simulink model "force_control_teaching_harness"  (R2016b)
settings: Solver=ode45  StartTime=0.0  StopTime=1  RelTol=1e-3  EnableMultiTasking=on
undefined symbols (not defined in the file): sigbuilder_block
settings Model: ModifiedByFormat=The MathWorks Inc.  Creator=The MathWorks, Inc.  LastModifiedBy=The MathWorks Inc.
settings DataIOCC: LimitDataPoints=on  SaveFormat=Array  SaveOutput=off  SaveTime=off
settings OptimizationCC: ExpressionDepthLimit=2147483647  LifeSpan=1
settings DebuggingCC: UnderspecifiedInitializationDetection=Classic  MergeDetectMultiDrivingBlocksExec=none  SolverPrmCheckMsg=warning  FcnCallInpInsideContextMsg=warning  StateNameClashWarn=warning  SFUnexpectedBacktrackingDiag=warning  SFNoUnconditionalDefaultTransitionDiag=warning  SFExecutionAtInitializationDiag=none
settings HardwareCC: ProdBitPerPointer=32  ProdBitPerSizeT=32  ProdBitPerPtrDiffT=32  ProdLargestAtomicFloat=None  ProdIntDivRoundTo=Undefined  ProdEndianess=Unspecified  ProdWordSize=32  ProdHWDeviceType=32-bit Generic
settings ModelReferenceCC: PropagateSignalLabelsOutOfModel=off
settings GRTTargetCC: TargetLangStandard=C89/C90 (ANSI)  GeneratePreprocessorConditionals=Disable all  CombineOutputUpdateFcns=off  GRTInterface=on
settings ConfigComp: CovMetricSettings=dw  CovHtmlReporting=on  CovSaveCumulativeToWorkspaceVar=on  CovSaveSingleToWorkspaceVar=on  CovExternalEMLEnable=off  CovSFcnEnable=off

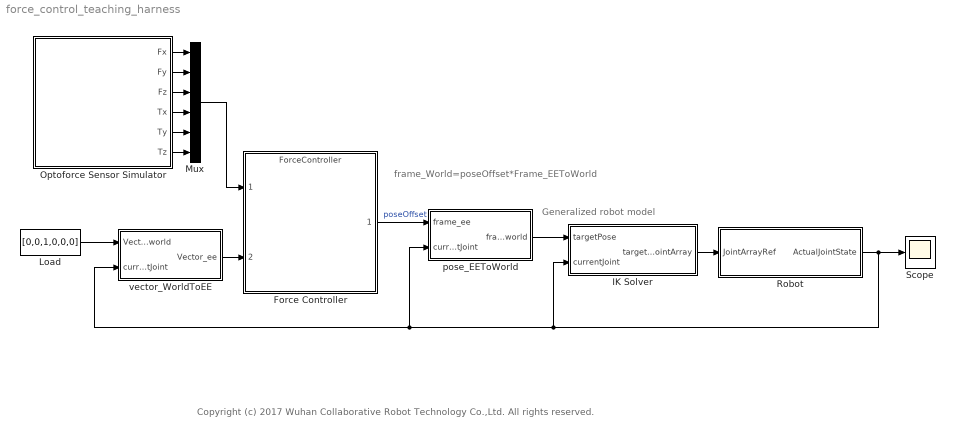
== system force_control_teaching_harness ==
  note: frame_World=poseOffset*Frame_EEToWorld
  note: Generalized robot model
  note: Copyright (c) 2017 Wuhan Collaborative Robot Technology Co.,Ltd. All rights reserved.
  Force Controller : ModelReference  ModelNameDialog=ForceController.slx  SimulationMode=Normal  ModelReferenceVersion=1.135
  IK Solver : Subsystem
  Load : Constant  Value=[0,0,1,0,0,0]
  Mux : Mux  Inputs=6
  Optoforce Sensor Simulator : Subsystem  Tag=STV Subsys  LoadFcn=sigbuilder_block('load');  StartFcn=sigbuilder_block('start');  StopFcn=sigbuilder_block('stop');  ClipboardFcn=sigbuilder_block('clipboard');  mask(Sigbuilder block){tuvar=[0:10]}
      mask help: Simulink:masks:SigbuilderBlock_MD
      mask init:
      | if ~strcmp(get_param(bdroot(gcbh),'SimulationStatus'),'stopped') tuvar = sigbuilder_block('maskInit'); end
      settings: CopyFcn=sigbuilder_block('copy');  DeleteFcn=sigbuilder_block('delete');  ModelCloseFcn=sigbuilder_block('modelClose');  PreSaveFcn=sigbuilder_block('preSave');  PauseFcn=sigbuilder_block('pause');  ContinueFcn=sigbuilder_block('continue');  NameChangeFcn=sigbuilder_block('namechange');  OpenFcn=sigbuilder_block('open',[6 30 1428 681 ]);  CloseFcn=sigbuilder_block('close');
      mask Display: plot(0, 0, 100, 100,[2, 2, 32, 32, 2], [68, 8, 8, 68, 68],[32, 2], [38, 38], [32, 19, 2],[53, 60, 44], [32, 17, 17, 2],[16, 16, 31, 31]);txt = getActiveGroup(gcbh);text(2, 100, txt,'verticalAlignment', 'top');
  Robot : Subsystem
  Scope : Scope
  pose_EEToWorld : Subsystem
  vector_WorldToEE : Subsystem
  wires:
  Optoforce Sensor Simulator/1(Fx) -> Mux/1
  Force Controller/1 -> pose_EEToWorld/1(frame_ee)  "poseOffset"
  Robot/1(ActualJointState) -> Scope/1, pose_EEToWorld/2(currentJoint), vector_WorldToEE/2(currentJoint), IK Solver/2(currentJoint)
  IK Solver/1(targetJointArray) -> Robot/1(JointArrayRef)
  Optoforce Sensor Simulator/2(Fy) -> Mux/2
  Optoforce Sensor Simulator/3(Fz) -> Mux/3
  Optoforce Sensor Simulator/4(Tx) -> Mux/4
  Optoforce Sensor Simulator/5(Ty) -> Mux/5
  Optoforce Sensor Simulator/6(Tz) -> Mux/6
  Mux/1 -> Force Controller/1
  Load/1 -> vector_WorldToEE/1(Vector_world)
  vector_WorldToEE/1(Vector_ee) -> Force Controller/2
  pose_EEToWorld/1(frame_world) -> IK Solver/1(targetPose)

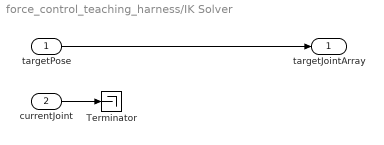
== system force_control_teaching_harness/IK Solver ==
  targetPose : Inport  PortDimensions=6
  currentJoint : Inport  Port=2  PortDimensions=6
  Terminator : Terminator
  targetJointArray : Outport
  wires:
  targetPose/1 -> targetJointArray/1
  currentJoint/1 -> Terminator/1

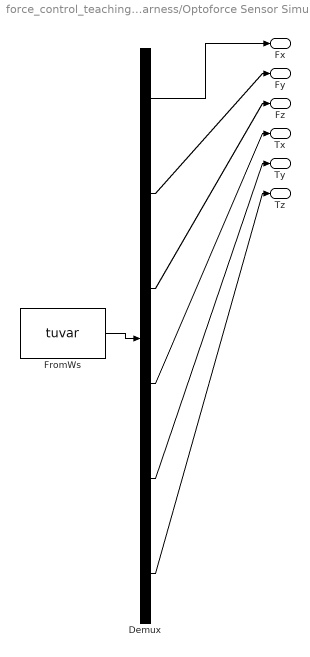
== system force_control_teaching_harness/Optoforce Sensor Simulator ==
  Demux : Demux  Tag=STV Demux  Outputs=6
  FromWs : FromWorkspace  Tag=STV FromWs  VariableName=tuvar  SampleTime=0
      SigBuilderData=|
      | common.afterFinalStr = 'Extrapolate'
      | common.sampleTime = 0
      | dataSet.timeRange = [0 10]
      | dataSet.name = 'Group 1'
      | sbobj.Groups.Name = 'Group 1'
      | sbobj.Groups.Signals(1).Name = 'Fx'
      | sbobj.Groups.Signals(1).XData = [0 4 4 6 6 10]
      | sbobj.Groups.Signals(1).YData = [0 0 1 1 0 0]
      | sbobj.Groups.Signals(2).Name = 'Fy'
      | sbobj.Groups.Signals(2).XData = [0 5 5 10]
      | sbobj.Groups.Signals(2).YData = [0 0 1 1]
      | sbobj.Groups.Signals(3).Name = 'Fz'
      | sbobj.Groups.Signals(3).XData = [0 5 5 10]
      | sbobj.Groups.Signals(3).YData = [0 0 1 1]
      | sbobj.Groups.Signals(4).Name = 'Tx'
      | sbobj.Groups.Signals(4).XData = [0 5 5 10]
      | sbobj.Groups.Signals(4).YData = [0 0 1 1]
      | sbobj.Groups.Signals(5).Name = 'Ty'
      | sbobj.Groups.Signals(5).XData = [0 5 5 10]
      | sbobj.Groups.Signals(5).YData = [0 0 1 1]
      | sbobj.Groups.Signals(6).Name = 'Tz'
      | sbobj.Groups.Signals(6).XData = [0 5 5 10]
      | sbobj.Groups.Signals(6).YData = [0.02 0.02 1 1]
  Fx : Outport  Tag=STV Outport
  Fy : Outport  Tag=STV Outport  Port=2
  Fz : Outport  Tag=STV Outport  Port=3
  Tx : Outport  Tag=STV Outport  Port=4
  Ty : Outport  Tag=STV Outport  Port=5
  Tz : Outport  Tag=STV Outport  Port=6
  wires:
  Demux/1 -> Fx/1
  FromWs/1 -> Demux/1
  Demux/2 -> Fy/1
  Demux/3 -> Fz/1
  Demux/4 -> Tx/1
  Demux/5 -> Ty/1
  Demux/6 -> Tz/1

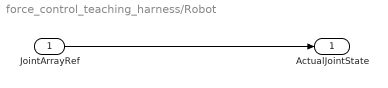
== system force_control_teaching_harness/Robot ==
  JointArrayRef : Inport  PortDimensions=6
  ActualJointState : Outport
  wires:
  JointArrayRef/1 -> ActualJointState/1

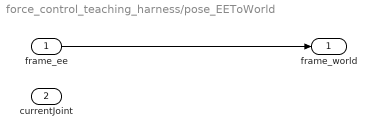
== system force_control_teaching_harness/pose_EEToWorld ==
  frame_ee : Inport  PortDimensions=6
  currentJoint : Inport  Port=2  PortDimensions=6
  frame_world : Outport
  wires:
  frame_ee/1 -> frame_world/1

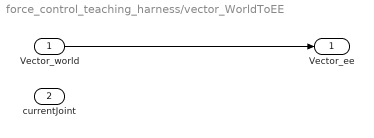
== system force_control_teaching_harness/vector_WorldToEE ==
  Vector_world : Inport  PortDimensions=6
  currentJoint : Inport  Port=2  PortDimensions=6
  Vector_ee : Outport
  wires:
  Vector_world/1 -> Vector_ee/1
